simulink library "slrtmotorlib"  (R2022b)
settings: Solver=VariableStepAuto  StartTime=0.0  StopTime=10.0  RelTol=1e-3
libraries: mcbhdllib x2
settings Model: Creator=chrisz  LastModifiedBy=chrisz
settings RTWCC: PlatformDefinition=Embedded Code

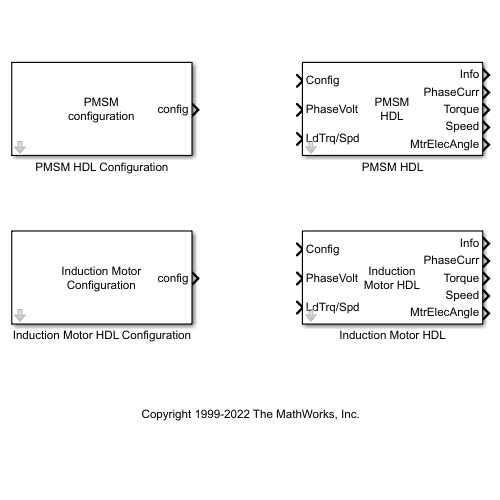
[thumbnail: Simulink's stored preview of the top-level diagram]
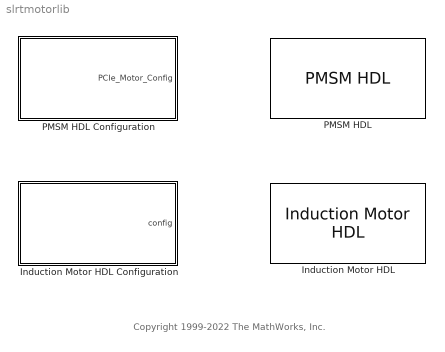
== system slrtmotorlib ==
  note: Copyright 1999-2022 The MathWorks, Inc.
  Induction Motor HDL : mcbhdllib/Electrical Systems/Motors/Induction Motor HDL  Ts=1e-6
  Induction Motor HDL Configuration : Subsystem  mask(Induction Motor Configuration){portConfig=Torque, Tw_mode=0, Ts=1e-6, P=2, Rs=1.77, Lls=0.0139, Rr=1.34, Llr=0.0121, Lm=0.3876, J=0.001, B=0, f=0}
      mask prompts: portConfig "Port configuration:"; Ts "Sample time (s):"; P "Number of pole pairs:"; Rs "Stator resistance (Ohm):"; Lls "Leakage inductance (H):"; Rr "Rotor resistance (Ohm):"; Llr "leakage inductance (H):"; Lm "Magnetizing inductance (H):"; J "Physical inertia (kg*m^2):"; B "viscous damping (N*m/rad/s):"; f "static friction (N*m):"
      mask help: Induction motor configuration block for HDL coder compatible implementation of induction motor block. This block intends to be used to configure the corresponding induction motor block on FPGA.
      settings: LibrarySourceBlock=mcbhdllib/Electrical Systems/Motors/Induction Motor Configuration
      mask TypeOptions portConfig: Torque | Speed
      mask Callback portConfig:
      | % Check the value selected in the pop-up
      | mask = Simulink.Mask.get(gcb);
      | portConfigStr = get_param(gcb, 'portConfig');
      | if strcmp(portConfigStr, 'Torque')
      |     % Set Tw_mode value to 0
      |     mask.getParameter('Tw_mode').Value = '0';
      | 
      | elseif strcmp(portConfigStr, 'Speed')
      |     % Set Tw_mode value to 1
      |     mask.getParameter('Tw_mode').Value = '1';
      | 
      | end
      mask DialogControl Container5 Prompt: Block options
      mask DialogControl Container7 Prompt: Parameters
      mask Display:
      | disp('Induction Motor\nConfiguration');
      | port_label('output', 1, 'config')
  PMSM HDL : mcbhdllib/Electrical Systems/Motors/PMSM HDL  VariantControl=pmsmVariant==pmsmEnum.TorqueInput  Ts=1e-6
  PMSM HDL Configuration : Subsystem  mask(PMSM Configuration){portConfig=Torque, Trq_N_mode=0, Ts=1e-6, Pp=4, Rs=0.02, Ld=1.7e-3, Lq=3.2e-3, lambda_pm=0.2205, J=0.0027, B=4.924e-4, f=0}
      mask prompts: portConfig "Mechanical input configuration:"; Ts "Sample time (s):"; Pp "Number of pole pairs:"; Rs "Stator resistance per phase (Ohm):"; Ld "Stator d-axis inductance (H):"; Lq "Stator q-axis inductance (H):"; lambda_pm "Permanent magnet flux linkage (Wb):"; J "Inertia (kgm^2):"; B "Viscous damping (Nm/rad/s):"; f "Static friction (Nm):"
      mask help: PMSM configuration block for HDL coder compatible implementation of PMSM block. This block intends to be used to configure the corresponding PMSM block on FPGA.
      settings: LibrarySourceBlock=mcbhdllib/Electrical Systems/Motors/PMSM Configuration
      mask TypeOptions portConfig: Torque | Speed
      mask Callback portConfig:
      | % Check the value selected in the pop-up
      | mask = Simulink.Mask.get(gcb);
      | portConfigStr = get_param(gcb, 'portConfig');
      | if strcmp(portConfigStr, 'Torque')
      |     % Set Trq_N_mode value to 0
      |     mask.getParameter('Trq_N_mode').Value = '0';
      | 
      | elseif strcmp(portConfigStr, 'Speed')
      |     % Set Trq_N_mode value to 2
      |     mask.getParameter('Trq_N_mode').Value = '1';
      | 
      | end
      mask DialogControl ParameterGroupVar Prompt: Block options
      mask DialogControl Container4 Prompt: Parameters
      mask Display:
      | disp('PMSM\nconfiguration');
      | port_label('output',1,'config');

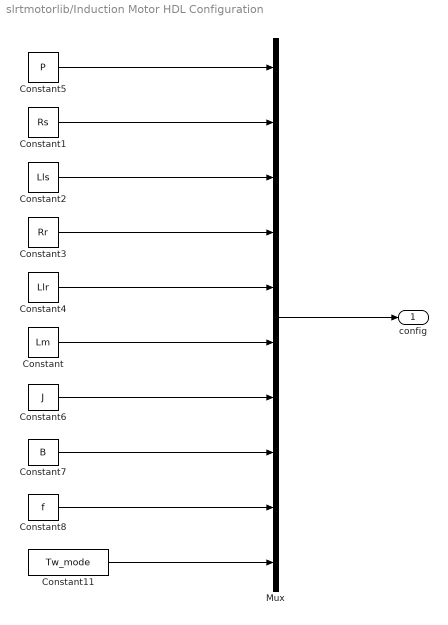
== system slrtmotorlib/Induction Motor HDL Configuration ==
  Constant : Constant  Value=Lm  OutDataTypeStr=single  SampleTime=Ts
  Constant1 : Constant  Value=Rs  OutDataTypeStr=single  SampleTime=Ts
  Constant11 : Constant  Value=Tw_mode  OutDataTypeStr=single  SampleTime=Ts
  Constant2 : Constant  Value=Lls  OutDataTypeStr=single  SampleTime=Ts
  Constant3 : Constant  Value=Rr  OutDataTypeStr=single  SampleTime=Ts
  Constant4 : Constant  Value=Llr  OutDataTypeStr=single  SampleTime=Ts
  Constant5 : Constant  Value=P  OutDataTypeStr=single  SampleTime=Ts
  Constant6 : Constant  Value=J  OutDataTypeStr=single  SampleTime=Ts
  Constant7 : Constant  Value=B  OutDataTypeStr=single  SampleTime=Ts
  Constant8 : Constant  Value=f  OutDataTypeStr=single  SampleTime=Ts
  Mux : Mux  Inputs=10
  config : Outport
  wires:
  Constant1/1 -> Mux/2
  Constant2/1 -> Mux/3
  Constant3/1 -> Mux/4
  Constant4/1 -> Mux/5
  Constant6/1 -> Mux/7
  Constant7/1 -> Mux/8
  Constant8/1 -> Mux/9
  Mux/1 -> config/1
  Constant11/1 -> Mux/10
  Constant5/1 -> Mux/1
  Constant/1 -> Mux/6

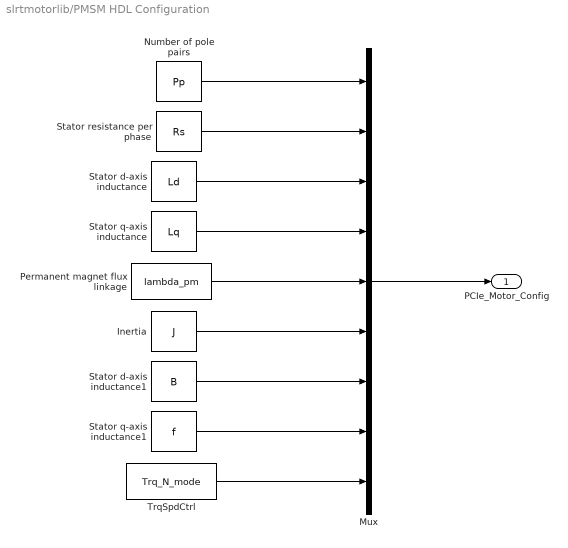
== system slrtmotorlib/PMSM HDL Configuration ==
  Inertia : Constant  Value=J  OutDataTypeStr=single  SampleTime=Ts
  Mux : Mux  Inputs=9
  Number of pole pairs : Constant  Value=Pp  OutDataTypeStr=single  SampleTime=Ts
  Permanent magnet flux linkage : Constant  Value=lambda_pm  OutDataTypeStr=single  SampleTime=Ts
  Stator d-axis inductance : Constant  Value=Ld  OutDataTypeStr=single  SampleTime=Ts
  Stator d-axis inductance1 : Constant  Value=B  OutDataTypeStr=single  SampleTime=Ts
  Stator q-axis inductance : Constant  Value=Lq  OutDataTypeStr=single  SampleTime=Ts
  Stator q-axis inductance1 : Constant  Value=f  OutDataTypeStr=single  SampleTime=Ts
  Stator resistance per phase : Constant  Value=Rs  OutDataTypeStr=single  SampleTime=Ts
  TrqSpdCtrl : Constant  Value=Trq_N_mode  OutDataTypeStr=single  SampleTime=Ts
  PCIe_Motor_Config : Outport
  wires:
  Number of pole pairs/1 -> Mux/1
  Stator d-axis inductance/1 -> Mux/3
  Stator q-axis inductance/1 -> Mux/4
  Inertia/1 -> Mux/6
  Mux/1 -> PCIe_Motor_Config/1
  Stator d-axis inductance1/1 -> Mux/7
  Stator q-axis inductance1/1 -> Mux/8
  TrqSpdCtrl/1 -> Mux/9
  Stator resistance per phase/1 -> Mux/2
  Permanent magnet flux linkage/1 -> Mux/5
